simulink model "Embedded_Model_itworks"  (R2024a)
settings: Solver=FixedStepDiscrete  StartTime=0.0  StopTime=Inf  FixedStep=0.002  RelTol=1e-3  EnableMultiTasking=on
values from neighbouring files (symbols this model uses):
  theta_hip_rad = [0 5e-06 2.2e-05 4.9e-05 8.8e-05 0.000137 0.000197 0.000268 0.000349 0.000441 0.000545 0.000657 ... (1200 elements, 1x1200)]    [target_theta_vector.mat]
  theta_knee_rad = [0 -1.2e-05 -4.9e-05 -0.00011 -0.000196 -0.000304 -0.000438 -0.000596 -0.000776 -0.00098 -0.001209 -0.001459 ... (1200 elements, 1x1200)]    [target_theta_vector.mat]
  theta_l1_rad = [0 0 0 0 0 0 0 0 0 0 0 0 ... (1200 elements, 1x1200)]    [target_theta_vector.mat]
undefined symbols (not defined in the file or in its folder): Down, GPTRIP1SEL, TZ1, Up
libraries: c280xlib x10, c2000lib x1, c2837xDlib x1, slpidlib x1, c2802xlib x1
settings Model: ExtModeTrigDuration=8  Creator=The MathWorks, Inc.  LastModifiedBy=wnsgh
settings SolverCC: AllowMultiTaskInputOutput=on  AlgebraicLoopSolver=TrustRegion  AutoInsertRateTranBlk=on  MaxZcPerStep=1
settings OptimizationCC: DefaultUnderspecifiedDataType=single  EnhancedBackFolding=on  PassReuseOutputArgsAs=Individual arguments  MaxStackSize=1024  OptimizeBlockOrder=speed  DifferentSizesBufferReuse=on  OptimizationCustomize=off  DenormalBehavior=FlushToZero  EfficientTunableParamExpr=on
settings DebuggingCC: MultiTaskDSMMsg=none  ParameterTunabilityLossMsg=error  UnconnectedInputMsg=warning  UnconnectedOutputMsg=warning  UnconnectedLineMsg=warning
settings HardwareCC: ProdBitPerChar=16  ProdBitPerInt=16  ProdBitPerPointer=32  ProdBitPerSizeT=32  ProdBitPerPtrDiffT=32  ProdLargestAtomicInteger=Integer  ProdLargestAtomicFloat=None  ProdWordSize=16  ProdLongLongMode=on  ProdHWDeviceType=Texas Instruments->C2000
settings ModelReferenceCC: EnableRefExpFcnMdlSchedulingChecks=on
settings SFSimCC: MATLABDynamicMemAlloc=off
settings RTWCC: Description=Embedded Coder  SystemTargetFile=ert.tlc  HardwareBoard=TI Delfino F28379D LaunchPad  TemplateMakefile=ert_default_tmf  GenerateReport=on  Toolchain=Texas Instruments Code Composer Studio (C2000)  GPUComputeCapability=3.5  DLArmComputeVersion=19.05
settings CodeAppCC: ForceParamTrailComments=on  IgnoreCustomStorageClasses=off  OperatorAnnotations=on  SimulinkDataObjDesc=on  SFDataObjDesc=on  InsertBlockDesc=on
settings ERTTargetCC: CodeReplacementLibrary=TI C28x  ExtModeStaticAllocSize=10000

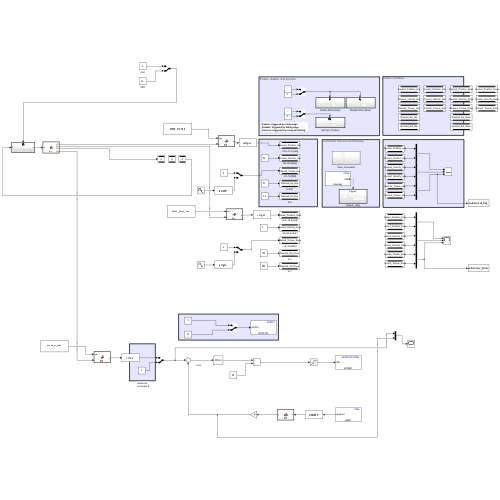
[thumbnail: Simulink's stored preview of the top-level diagram]
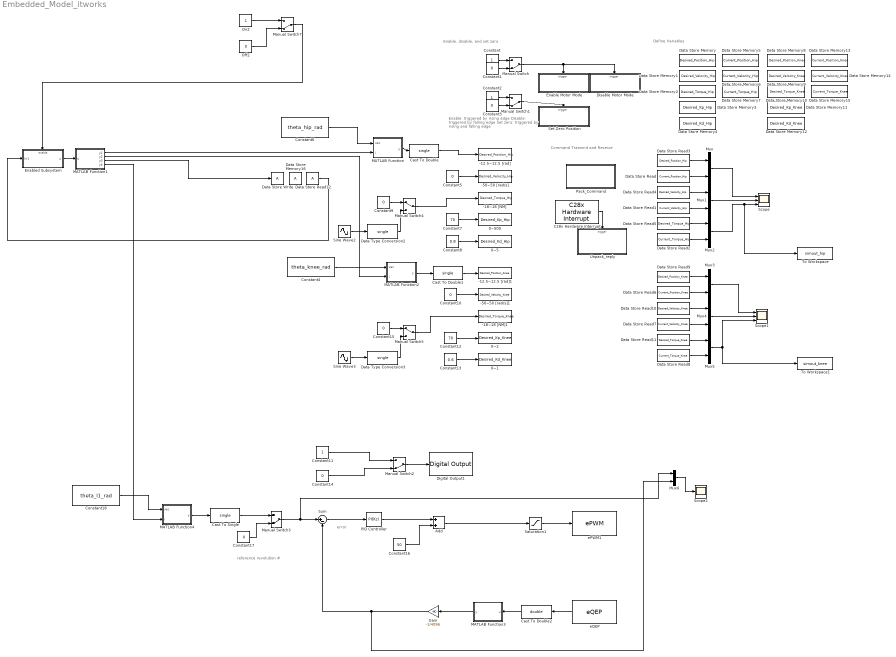
== system Embedded_Model_itworks ==
  note: Enable: triggered by rising edge
      | Disable: triggered by falling edge
      | Set zero: triggered by rising and falling edge
  note: Define Variables
  note: Enable, disable, and set zero
  note: Command Transmit and Receive
  note: reference
      | revolution #
  note: error
  -12.5~12.5 [rad] : DataStoreWrite  DataStoreName=Desired_Position_Hip  IndexOptions=Index vector (dialog)  Indices=1  OutputSizes=1
  -12.5~12.5 [rad]1 : DataStoreWrite  DataStoreName=Desired_Position_Knee  IndexOptions=Index vector (dialog)  Indices=1  OutputSizes=1
  -18~18 [NM] : DataStoreWrite  DataStoreName=Desired_Torque_Hip  IndexOptions=Index vector (dialog)  Indices=1  OutputSizes=1
  -18~18 [NM]1 : DataStoreWrite  DataStoreName=Desired_Torque_Knee  IndexOptions=Index vector (dialog)  Indices=1  OutputSizes=1
  -50~50 [rad/s] : DataStoreWrite  DataStoreName=Desired_Velocity_Hip  IndexOptions=Index vector (dialog)  Indices=1  OutputSizes=1
  -50~50 [rad/s]1 : DataStoreWrite  DataStoreName=Desired_Velocity_Knee  IndexOptions=Index vector (dialog)  Indices=1  OutputSizes=1
  0~1 : DataStoreWrite  DataStoreName=Desired_Kd_Knee  IndexOptions=Index vector (dialog)  Indices=1  OutputSizes=1
  0~2 : DataStoreWrite  DataStoreName=Desired_Kp_Knee  IndexOptions=Index vector (dialog)  Indices=1  OutputSizes=1
  0~5 : DataStoreWrite  DataStoreName=Desired_Kd_Hip  IndexOptions=Index vector (dialog)  Indices=1  OutputSizes=1
  0~500 : DataStoreWrite  DataStoreName=Desired_Kp_Hip  IndexOptions=Index vector (dialog)  Indices=1  OutputSizes=1
  Add : Sum
  C28x Hardware Interrupt : c2000lib/Scheduling/C28x Hardware Interrupt  irqnumbers=[9]  pienumbers=[8]  irqpriorities=[30]  irqpreempts=[1]  showinput=off  dspchiptype=C280X
  Cast To Double : DataTypeConversion  OutDataTypeStr=single  SaturateOnIntegerOverflow=off  RndMeth=Floor
  Cast To Double1 : DataTypeConversion  OutDataTypeStr=single  SaturateOnIntegerOverflow=off  RndMeth=Floor
  Cast To Double2 : DataTypeConversion  OutDataTypeStr=double  SaturateOnIntegerOverflow=off  RndMeth=Floor
  Cast To Single : DataTypeConversion  OutDataTypeStr=single  SaturateOnIntegerOverflow=off  RndMeth=Floor
  Constant : Constant
  Constant{1,3,14,17} (4 alike) : Constant  Value=0
  Constant{5,9..10,15} (4 alike) : Constant  Value=0  OutDataTypeStr=single
  Constant11 : Constant
  Constant12 : Constant  Value=70  OutDataTypeStr=single
  Constant13 : Constant  Value=0.6  OutDataTypeStr=single
  Constant16 : Constant  Value=50
  Constant18 : Constant  Value=theta_l1_rad
  Constant2 : Constant
  Constant4 : Constant  Value=theta_knee_rad
  Constant6 : Constant  Value=theta_hip_rad
  Constant7 : Constant  Value=70  OutDataTypeStr=single
  Constant8 : Constant  Value=0.8  OutDataTypeStr=single
  Data Store Memory : DataStoreMemory  DataStoreName=Desired_Position_Hip  WriteAfterWriteMsg=warning  ShowAdditionalParam=off  OutDataTypeStr=single
  Data Store Memory1 : DataStoreMemory  DataStoreName=Desired_Velocity_Hip  WriteAfterWriteMsg=warning  ShowAdditionalParam=off  OutDataTypeStr=single
  Data Store Memory10 : DataStoreMemory  DataStoreName=Desired_Torque_Knee  WriteAfterWriteMsg=warning  ShowAdditionalParam=off  OutDataTypeStr=single
  Data Store Memory11 : DataStoreMemory  DataStoreName=Desired_Kp_Knee  WriteAfterWriteMsg=warning  ShowAdditionalParam=off  OutDataTypeStr=single
  Data Store Memory12 : DataStoreMemory  DataStoreName=Desired_Kd_Knee  WriteAfterWriteMsg=warning  ShowAdditionalParam=off  OutDataTypeStr=single
  Data Store Memory13 : DataStoreMemory  DataStoreName=Current_Position_Knee  WriteAfterWriteMsg=warning  ShowAdditionalParam=off  OutDataTypeStr=single
  Data Store Memory14 : DataStoreMemory  DataStoreName=Current_Velocity_Knee  WriteAfterWriteMsg=warning  ShowAdditionalParam=off  OutDataTypeStr=single
  Data Store Memory15 : DataStoreMemory  DataStoreName=Current_Torque_Knee  WriteAfterWriteMsg=warning  ShowAdditionalParam=off  OutDataTypeStr=single
  Data Store Memory16 : DataStoreMemory  WriteAfterWriteMsg=warning  ShowAdditionalParam=off
  Data Store Memory2 : DataStoreMemory  DataStoreName=Desired_Torque_Hip  WriteAfterWriteMsg=warning  ShowAdditionalParam=off  OutDataTypeStr=single
  Data Store Memory3 : DataStoreMemory  DataStoreName=Desired_Kp_Hip  WriteAfterWriteMsg=warning  ShowAdditionalParam=off  OutDataTypeStr=single
  Data Store Memory4 : DataStoreMemory  DataStoreName=Desired_Kd_Hip  WriteAfterWriteMsg=warning  ShowAdditionalParam=off  OutDataTypeStr=single
  Data Store Memory5 : DataStoreMemory  DataStoreName=Current_Position_Hip  WriteAfterWriteMsg=warning  ShowAdditionalParam=off  OutDataTypeStr=single
  Data Store Memory6 : DataStoreMemory  DataStoreName=Current_Velocity_Hip  WriteAfterWriteMsg=warning  ShowAdditionalParam=off  OutDataTypeStr=single
  Data Store Memory7 : DataStoreMemory  DataStoreName=Current_Torque_Hip  WriteAfterWriteMsg=warning  ShowAdditionalParam=off  OutDataTypeStr=single
  Data Store Memory8 : DataStoreMemory  DataStoreName=Desired_Position_Knee  WriteAfterWriteMsg=warning  ShowAdditionalParam=off  OutDataTypeStr=single
  Data Store Memory9 : DataStoreMemory  DataStoreName=Desired_Velocity_Knee  WriteAfterWriteMsg=warning  ShowAdditionalParam=off  OutDataTypeStr=single
  Data Store Read : DataStoreRead  DataStoreName=Current_Position_Hip  IndexOptions=Index vector (dialog)  Indices=1  OutputSizes=1
  Data Store Read1 : DataStoreRead  DataStoreName=Current_Velocity_Hip  IndexOptions=Index vector (dialog)  Indices=1  OutputSizes=1
  Data Store Read10 : DataStoreRead  DataStoreName=Desired_Velocity_Knee  IndexOptions=Index vector (dialog)  Indices=1  OutputSizes=1
  Data Store Read11 : DataStoreRead  DataStoreName=Desired_Torque_Knee  IndexOptions=Index vector (dialog)  Indices=1  OutputSizes=1
  Data Store Read12 : DataStoreRead  IndexOptions=Index vector (dialog)  Indices=1  OutputSizes=1
  Data Store Read2 : DataStoreRead  DataStoreName=Current_Torque_Hip  IndexOptions=Index vector (dialog)  Indices=1  OutputSizes=1
  Data Store Read3 : DataStoreRead  DataStoreName=Desired_Position_Hip  IndexOptions=Index vector (dialog)  Indices=1  OutputSizes=1
  Data Store Read4 : DataStoreRead  DataStoreName=Desired_Velocity_Hip  IndexOptions=Index vector (dialog)  Indices=1  OutputSizes=1
  Data Store Read5 : DataStoreRead  DataStoreName=Desired_Torque_Hip  IndexOptions=Index vector (dialog)  Indices=1  OutputSizes=1
  Data Store Read6 : DataStoreRead  DataStoreName=Current_Position_Knee  IndexOptions=Index vector (dialog)  Indices=1  OutputSizes=1
  Data Store Read7 : DataStoreRead  DataStoreName=Current_Velocity_Knee  IndexOptions=Index vector (dialog)  Indices=1  OutputSizes=1
  Data Store Read8 : DataStoreRead  DataStoreName=Current_Torque_Knee  IndexOptions=Index vector (dialog)  Indices=1  OutputSizes=1
  Data Store Read9 : DataStoreRead  DataStoreName=Desired_Position_Knee  IndexOptions=Index vector (dialog)  Indices=1  OutputSizes=1
  Data Store Write : DataStoreWrite  IndexOptions=Index vector (dialog)  Indices=1  OutputSizes=1
  Data Type Conversion2 : DataTypeConversion  OutDataTypeStr=single  SaturateOnIntegerOverflow=off  RndMeth=Floor
  Data Type Conversion3 : DataTypeConversion  OutDataTypeStr=single  SaturateOnIntegerOverflow=off  RndMeth=Floor
  Digital Output1 : c2837xDlib/Digital Output  GPIO_Number=GPIO0~GPIO7  GPIO_Bit0=off  GPIO_BIT0_Toggle=off  GPIO_Bit1=off  GPIO_BIT1_Toggle=off  GPIO_Bit2=off  GPIO_BIT2_Toggle=off  GPIO_Bit3=on  GPIO_BIT3_Toggle=off  GPIO_Bit4=off  GPIO_BIT4_Toggle=off  GPIO_Bit5=off  GPIO_BIT5_Toggle=off  GPIO_Bit6=off  GPIO_BIT6_Toggle=off  GPIO_Bit7=off  GPIO_BIT7_Toggle=off
  Disable Motor Mode : Subsystem
  Enable Motor Mode : Subsystem
  Enabled Subsystem : Subsystem  TreatAsAtomicUnit=on
  Gain : Gain  Gain=-1/4096
  MATLAB Function : MATLAB Function  TreatAsAtomicUnit=on
  MATLAB Function1 : MATLAB Function  TreatAsAtomicUnit=on
  MATLAB Function2 : MATLAB Function  TreatAsAtomicUnit=on
  MATLAB Function3 : MATLAB Function  TreatAsAtomicUnit=on
  MATLAB Function4 : MATLAB Function  TreatAsAtomicUnit=on
  Manual Switch{,1..3,7} (5 alike) : ManualSwitch  CurrentSetting=0
  Manual Switch4 : ManualSwitch
  Manual Switch5 : ManualSwitch
  Mux{,1..6} (7 alike) : Mux  Inputs=2
  Off2 : Constant  Value=0
  On2 : Constant
  PID Controller : slpidlib/PID Controller  Controller=PID  Form=Parallel  TimeDomain=Discrete-time  UseExternalTs=off  SampleTime=-1  IntegratorMethod=Forward Euler  FilterMethod=Forward Euler  ControllerParametersSource=internal  P=70  I=5  UseKiTs=off  D=2  UseExternalDerivativeSource=off  N=100  UseFilter=on  TunerSelectOption=Frequency Response Based  InitialConditionSource=internal  InitialConditionForIntegrator=0  InitialConditionForFilter=0  DifferentiatorICPrevScaledInput=0  ExternalReset=none  TrackingMode=off  Kt=1  LimitOutput=off  SatLimitsSource=internal  UpperSaturationLimit=inf  LowerSaturationLimit=-inf  LinearizeAsGain=on  AntiWindupMode=none  Kb=1  LimitIntegrator=off  UpperIntegratorSaturationLimit=inf  LowerIntegratorSaturationLimit=-inf  POutMin=[]  POutMax=[]  IOutMin=[]  IOutMax=[]  DOutMin=[]  DOutMax=[]  NOutMin=[]  NOutMax=[]  SumOutMin=[]  SumOutMax=[]  SaturationOutMin=[]  SaturationOutMax=[]  PParamMin=[]  PParamMax=[]  IParamMin=[]  IParamMax=[]  DParamMin=[]  DParamMax=[]  NParamMin=[]  NParamMax=[]  KbParamMin=[]  KbParamMax=[]  KtParamMin=[]  KtParamMax=[]  KbOutMin=[]  KbOutMax=[]  KtOutMin=[]  KtOutMax=[]  IntegratorOutMin=[]  IntegratorOutMax=[]  FilterOutMin=[]  FilterOutMax=[]  SumI1OutMin=[]  SumI1OutMax=[]  SumI2OutMin=[]  SumI2OutMax=[]  SumI3OutMin=[]  SumI3OutMax=[]  SumI4OutMin=[]  SumI4OutMax=[]  SumDOutMin=[]  SumDOutMax=[]  DifferentiatorOutMin=[]  DifferentiatorOutMax=[]  FilterDiffOutCoefMin=[]  FilterDiffOutCoefMax=[]  ReciprocalOutMin=[]  ReciprocalOutMax=[]  SumDenOutMin=[]  SumDenOutMax=[]  SumNumOutMin=[]  SumNumOutMax=[]  DivideOutMin=[]  DivideOutMax=[]  UdiffTsProdOutMin=[]  UdiffTsProdOutMax=[]  NTsProdOutMin=[]  NTsProdOutMax=[]  UintegralTsProdOutMin=[]  UintegralTsProdOutMax=[]  UngainTsProdOutMin=[]  UngainTsProdOutMax=[]  ClampingZeroOutDataTypeStr=Inherit: Inherit via back propagation  ClampingZeroOutMin=[]  ClampingZeroOutMax=[]  FilterDenConstantOutDataTypeStr=Inherit: Inherit via back propagation  FilterDenConstantOutMin=[]  FilterDenConstantOutMax=[]  PCopyOutDataTypeStr=Inherit: Inherit via back propagation  PCopyOutMin=[]  PCopyOutMax=[]  NCopyOutDataTypeStr=Inherit: Inherit via back propagation  NCopyOutMin=[]  NCopyOutMax=[]  IntegratorContinuousStateAttributes=''  IntegratorStateMustResolveToSignalObject=off  IntegratorRTWStateStorageClass=Auto  FilterContinuousStateAttributes=''  FilterStateMustResolveToSignalObject=off  FilterRTWStateStorageClass=Auto  ParallelPVariant=InternalParameters  IdealPVariant=Disabled  IVariant=InternalParameters  DVariant=InternalParameters  IntegratorVariant=Discrete  SatVariant=Disabled  AWVariant=Passthrough  PCopyVariant=Disabled  TRVariant=Disabled  FdbkBlocksVariant=Forward  IdealPFdbkVariant=Disabled  SatFdbkVariant=Disabled  DerivativeFilterVariant=ForwardEulerFilter  NVariant=InternalParameters  NCopyVariant=Disabled  FilterICVariant=InternalICsFilter  IntegratorICVariant=InternalICs  ExternalResetVariant=Disabled  TRSumVariant=Passthrough  SumFdbkVariant=Disabled  SumVariant=Sum_PID  TsampFilterVariant=InternalTs  TsampNgainVariant=Passthrough  TsampIntegralVariant=Disabled_SignalSpec  ExternalSaturationOutDataTypeStr=Inherit: Same as second input  DerivativeSourceVariant=ErrorSignal
  Pack_Command : Subsystem
  Saturation1 : Saturate  UpperLimit=90  LowerLimit=10
  Scope : Scope  NumInputPorts=3
  Scope1 : Scope  NumInputPorts=3
  Scope2 : Scope
  Set Zero Position : Subsystem
  Sine Wave2 : Sin  Amplitude=0.5  Frequency=2*pi
  Sine Wave3 : Sin  Amplitude=0.5  Frequency=2*pi
  Sum : Sum  Inputs=|+-
  To Workspace : ToWorkspace  VariableName=simout_hip  SampleTime=-1
      settings: Save2DSignal=2-D array (concatenate along first dimension)
  To Workspace1 : ToWorkspace  VariableName=simout_knee  SampleTime=-1
      settings: Save2DSignal=2-D array (concatenate along first dimension)
  Unpack_reply : Subsystem  ScheduleAs=Aperiodic partition  PartitionName=Unpack_reply
  ePWM1 : c2802xlib/ePWM  PwmType=C2000_Type4  useModule=ePWM1  ePWMxLINKTBPRD=Not Linked  periodUnits=Seconds  timerSource=Specify via dialog  timerPeriod_clk=64000  timerPeriod_sec=0.0001  tbshadow=Counter equals to zero  countingMode=Up-Down  phaseActiveEnable=Disable  phaseDirection=Count down after sync  phaseActive=0  synchronizationEnable=off  dcaevt1Sync=off  dcbevt1Sync=off  synchronizationOption=Disable  dcbevt1SyncOut=off  dcaevt1SyncOut=off  cmpdSyncOut=off  cmpcSyncOut=off  cmpbSyncOut=off  zeroSyncOut=off  swfSyncOut=off  perSynchronizationOption=Counter equals to period (CTR=PRD)  clockPrescale=1  HSclockPrescale=1  enswap=off  ePWMxAStatus=on  ePWMxAactionLogic1=Set  ePWMxAactionLogic2=Clear  ePWMxAactionLogic3=Clear  ePWMxAactionLogic4=Set  ePWMxAactionLogic5=Do nothing  ePWMxAactionLogic6=Do nothing  ePWMxACSFenable=off  ePWMxACSFvalue=Forcing disable  ePWMxASFreload=Zero  ePWMxBStatus=off  ePWMxBactionLogic1=Set  ePWMxBactionLogic2=Clear  ePWMxBactionLogic3=Do nothing  ePWMxBactionLogic4=Do nothing  ePWMxBactionLogic5=Clear  ePWMxBactionLogic6=Set  ePWMxBCSFenable=off  ePWMxBCSFvalue=Forcing disable  ePWMxBSFreload=Zero  ePWNxBOutWay=off  ePWMxLINKCMPA=Not Linked  CMPAUnits=Percentages  CMPASource=Input port  CMPAValue_per=50  CMPAValue_clk=32000  enCMPAshadow=Counter equals to zero (CTR=Zero)  ePWMxLINKCMPB=Not Linked  CMPBUnits=Percentages  CMPBSource=Specify via dialog  CMPBValue_per=50  CMPBValue_clk=32000  enCMPBshadow=Counter equals to zero (CTR=Zero)  ePWMxLINKCMPC=Not Linked  CMPCUnits=Clock cycles  CMPCSource=Specify via dialog  CMPCValue_per=50  CMPCValue_clk=32000  enCMPCshadow=Counter equals to zero (CTR=Zero)  ePWMxLINKCMPD=Not Linked  CMPDUnits=Clock cycles  CMPDSource=Specify via dialog  CMPDValue_per=50  CMPDValue_clk=32000  enCMPDshadow=Counter equals to zero (CTR=Zero)  enableDBePWMxA=off  enableDBePWMxB=off  enhalfcycle=off  DBpolarity=Active high (AH)  DBedgeDelay=Positive  DBSource_ePWMxA=ePWMxA  DBSource_ePWMxB=ePWMxA  DBPeriodUnits=Clock cycles  DBperiodSource=Specify via dialog  REDperiod=0  FEDperiod=0  REDperiod_sec=0  FEDperiod_sec=0  LoadModeDBRED=Immediate without using shadow  LoadModeDBFED=Immediate without using shadow  adcstartModuleA=off  adcrequestEventA=First event  adcstartEventA=Digital Compare Module A Event 1 start of conversion (DCAEVT1.soc)  adcstartEventA_type2=Counter equals to zero (CTR=Zero)  adcstartModuleB=off  adcrequestEventB=First event  adcstartEventB=Counter equals to zero (CTR=Zero)  adcstartEventB_type2=Counter equals to zero (CTR=Zero)  intEn=off  intPrd=First event  intSel=Counter equals to zero (CTR=Zero)  intSel_type2=Counter equals to zero (CTR=Zero)  hrpe=off  enHRPWM=off  HRPWM_LoadMode=Counter equals to period (CTR=PRD)  HRPWM_CTLMode=Duty or Period control mode  HRPWM_EDGMode=Both edge  hrpeb=off  enHRPWMB=off  HRPWM_LoadModeB=Counter equals to zero (CTR=ZERO)  HRPWM_CTLModeB=Duty or Period control mode  HRPWM_EDGModeB=Both edge  enHRDBRED=off  enHRDBFED=off  enSFO=on  enautoconv=on  chopperEnable=off  chopperFrequency=1  chopperFirstwidth=1  chopperDuty=12.5%  tripZonesource=Specify via dialog  tzselOSHT1=off  tzselOSHT2=off  tzselOSHT3=off  tzselOSHT4=off  tzselOSHT5=off  tzselOSHT6=off  tzselOSHDCAEV1=off  tzselOSHDCBEV1=off  tzselCBC1=off  tzselCBC2=off  tzselCBC3=off  tzselCBC4=off  tzselCBC5=off  tzselCBC6=off  tzselCBCDCAEV2=off  tzselCBCDCBEV2=off  enTzOstIntr=off  enTzCbcIntr=off  enTzDCAEVT1Intr=off  enTzDCAEVT2Intr=off  enTzDCBEVT1Intr=off  enTzDCBEVT2Intr=off  tzclrCBCLatch=Counter equals to zero (CTR=Zero)  ePWMxAforced=No action  ePWMxBforced=No action  DCAEVT1forced=No action  DCBEVT1forced=No action  DCAEVT2forced=No action  DCBEVT2forced=No action  dcah=Trip Zone 1 input (TZ1)  dcal=Trip Zone 2 input (TZ2)  dcbh=Trip Zone 1 input (TZ1)  dcbl=Trip Zone 2 input (TZ2)  dcah_type2=GPTRIP1SEL/(TZ1)  dcal_type2=GPTRIP1SEL/(TZ1)  dcbh_type2=GPTRIP1SEL/(TZ1)  dcbl_type2=GPTRIP1SEL/(TZ1)  gendcaevt1=Event disabled  gendcaevt2=Event disabled  gendcbevt1=Event disabled  gendcbevt2=Event disabled  dcaevt1src=DCAEVT1 with sync  dcaevt2src=DCAEVT2 with sync  dcbevt1src=DCBEVT1 with sync  dcbevt2src=DCBEVT2 with sync  pulsesel=Counter equals to zero (CTR=Zero)  blankinv=off  blankoffset=0  blankwidth=0  evsrcsel=Filtered version of DCAEVT1 (DCAEVT1FILT)  encape=off
      settings: LibrarySourceBlock=c2837xDlib/ePWM
  eQEP : c280xlib/eQEP  useModule=eQEP1  pcInputmode=Quadrature-count  externalClockrate=2x resolution: Count the rising/falling edge  swapPolarityselection=Clockwise  qdfOutputport=off  qapPolarityselection=off  qbpPolarityselection=off  qipPolarityselection=off  qspPolarityselection=off  igatePolarityselection=off  sampleTime=-1  pcOutputport=on  pcMaximumvalue=2^24  indexInitializationcheck=off  indexInitializationevent=Rising edge  strobeInitializationcheck=off  strobeInitializationevent=Rising edge  softwareInitializationcheck=off  softwareInitializationsource=Set to init value at start up  softwareInitializationmode=on  pcInitialvalue=2147483648  pcResetmode=Reset on an index event  ieloutputport=off  indexEventlatch=Rising edge  seloutputport=off  strobeEventlatch=Rising edge  pcefOutputport=off  enableEqepcapture=off  qctmrOutputport=off  qcprdOutputport=off  captureTimerprescaler=128  upEventprescaler=128  overflowErrorflag=off  directionErrorflag=off  captureTimerposition=On position counter read  unitTimerperiod=100000000  captureTimerlatch=off  capturePeriodlatch=off  positionCounterlatch=off  soenPolarityselection=off  spselPolarityselection=Index pin is used for sync output  compareValuesource=Specify via dialog  shadowMode=Load on QPOSCNT=0  compareValue=4294967295  syncOutputwidth=1  polaritySyncoutput=Active high  watchdogEnable=off  watchdogTimer=65535  outport1Datatype=auto  outport2Datatype=auto  outport3Datatype=auto  outport4Datatype=auto  outport5Datatype=auto  outport6Datatype=auto  outport7Datatype=auto  outport8Datatype=auto  outport9Datatype=auto  outport10Datatype=auto  outport11Datatype=auto  outport12Datatype=auto  eqepinterrupt_pce=off  eqepinterrupt_qpe=off  eqepinterrupt_qdc=off  eqepinterrupt_wto=off  eqepinterrupt_pcu=off  eqepinterrupt_pco=off  eqepinterrupt_pcr=off  eqepinterrupt_pcm=off  eqepinterrupt_sel=off  eqepinterrupt_iel=off  eqepinterrupt_uto=off  pheOutputport=off  watchdogOutputport=off  outport13Datatype=auto  outport14Datatype=auto
      settings: LibrarySourceBlock=c2837xDlib/eQEP
  wires:
  Data Store Read9/1 -> Mux3/1
  Constant5/1 -> -50~50 [rad/s]/1
  Data Store Read8/1 -> Mux5/2
  Mux1/1 -> Scope/2
  Mux4/1 -> Scope1/2
  Data Store Read7/1 -> Mux4/2
  Constant13/1 -> 0~1/1
  Data Store Read10/1 -> Mux4/1
  Data Store Read11/1 -> Mux5/1
  Data Store Read6/1 -> Mux3/2
  Constant12/1 -> 0~2/1
  Mux5/1 -> To Workspace1/1, Scope1/3
  Constant2/1 -> Manual Switch1/1
  Mux2/1 -> To Workspace/1, Scope/3
  Constant/1 -> Manual Switch/1
  Data Store Read2/1 -> Mux2/2
  Data Store Read/1 -> Mux/2
  Data Store Read3/1 -> Mux/1
  Data Store Read5/1 -> Mux2/1
  Constant10/1 -> -50~50 [rad/s]1/1
  Data Store Read4/1 -> Mux1/1
  Constant7/1 -> 0~500/1
  Data Store Read1/1 -> Mux1/2
  Manual Switch1/1 -> Set Zero Position/Trigger
  Mux3/1 -> Scope1/1
  Constant3/1 -> Manual Switch1/2
  Manual Switch/1 -> Enable Motor Mode/Trigger, Disable Motor Mode/Trigger
  Constant1/1 -> Manual Switch/2
  Constant8/1 -> 0~5/1
  Mux/1 -> Scope/1
  C28x Hardware Interrupt/1 -> Unpack_reply/Trigger
  Sine Wave2/1 -> Data Type Conversion2/1
  Constant9/1 -> Manual Switch4/1
  Data Type Conversion2/1 -> Manual Switch4/2
  Constant15/1 -> Manual Switch5/1
  Data Type Conversion3/1 -> Manual Switch5/2
  Sine Wave3/1 -> Data Type Conversion3/1
  Manual Switch4/1 -> -18~18 [NM]/1
  Manual Switch5/1 -> -18~18 [NM]1/1
  MATLAB Function1/1(y1) -> MATLAB Function/2(i)
  MATLAB Function1/3(y3) -> Data Store Write/1
  Data Store Read12/1 -> Enabled Subsystem/1(In1)
  Enabled Subsystem/1(u) -> MATLAB Function1/1(u)
  Constant6/1 -> MATLAB Function/1(vec)
  Constant4/1 -> MATLAB Function2/1(vec)
  MATLAB Function1/2(y2) -> MATLAB Function2/2(i)
  MATLAB Function/1(y) -> Cast To Double/1
  Cast To Double/1 -> -12.5~12.5 [rad]/1
  MATLAB Function2/1(y) -> Cast To Double1/1
  Cast To Double1/1 -> -12.5~12.5 [rad]1/1
  Cast To Single/1 -> Manual Switch3/1
  Add/1 -> Saturation1/1
  Cast To Double2/1 -> MATLAB Function3/1(u)
  Saturation1/1 -> ePWM1/1
  PID Controller/1 -> Add/1
  Gain/1 -> Mux6/2, Sum/2
  Sum/1 -> PID Controller/1
  MATLAB Function3/1(y) -> Gain/1
  Manual Switch2/1 -> Digital Output1/1
  Constant14/1 -> Manual Switch2/2
  Constant17/1 -> Manual Switch3/2
  eQEP/1 -> Cast To Double2/1
  Manual Switch3/1 -> Mux6/1, Sum/1
  Constant16/1 -> Add/2
  Constant11/1 -> Manual Switch2/1
  Mux6/1 -> Scope2/1
  Constant18/1 -> MATLAB Function4/1(vec)
  MATLAB Function4/1(y) -> Cast To Single/1
  MATLAB Function1/4(y4) -> MATLAB Function4/2(i)
  On2/1 -> Manual Switch7/1
  Off2/1 -> Manual Switch7/2
  Manual Switch7/1 -> Enabled Subsystem/Enable

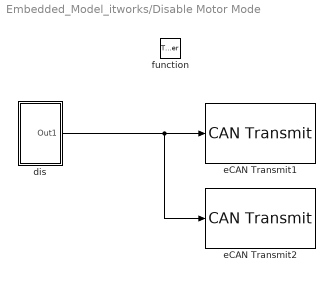
== system Embedded_Model_itworks/Disable Motor Mode ==
  function : TriggerPort  TriggerType=falling  VariantControl=(inherit)
  dis : Subsystem
  eCAN Transmit1 : c280xlib/CAN Transmit  chipFamily=C280x  useModule=CAN_B  mailboxNo=5  messageID=1  messageType=Standard (11-bit identifier)  enableBlockingMode=off  postInterrupt=off  interruptLine=0
  eCAN Transmit2 : c280xlib/CAN Transmit  chipFamily=C280x  useModule=CAN_B  mailboxNo=6  messageID=2  messageType=Standard (11-bit identifier)  enableBlockingMode=off  postInterrupt=off  interruptLine=0
  wires:
  dis/1(Out1) -> eCAN Transmit2/1, eCAN Transmit1/1

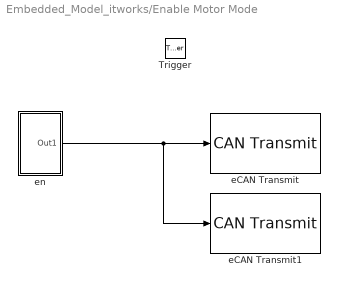
== system Embedded_Model_itworks/Enable Motor Mode ==
  Trigger : TriggerPort  VariantControl=(inherit)  PortDimensions=1
  eCAN Transmit : c280xlib/CAN Transmit  chipFamily=C280x  useModule=CAN_B  mailboxNo=3  messageID=1  messageType=Standard (11-bit identifier)  enableBlockingMode=off  postInterrupt=off  interruptLine=0
  eCAN Transmit1 : c280xlib/CAN Transmit  chipFamily=C280x  useModule=CAN_B  mailboxNo=4  messageID=2  messageType=Standard (11-bit identifier)  enableBlockingMode=off  postInterrupt=off  interruptLine=0
  en : Subsystem
  wires:
  en/1(Out1) -> eCAN Transmit1/1, eCAN Transmit/1

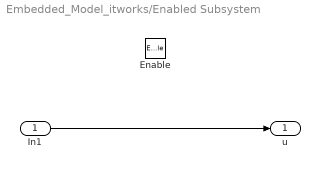
== system Embedded_Model_itworks/Enabled Subsystem ==
  In1 : Inport
  Enable : EnablePort
  u : Outport
  wires:
  In1/1 -> u/1

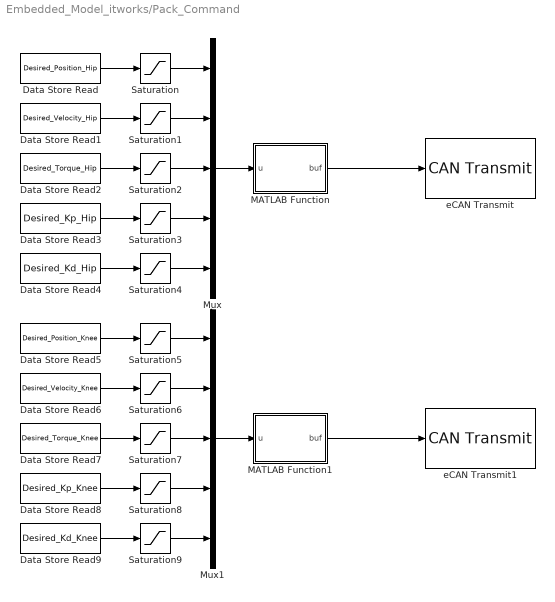
== system Embedded_Model_itworks/Pack_Command ==
  Data Store Read : DataStoreRead  DataStoreName=Desired_Position_Hip  IndexOptions=Index vector (dialog)  Indices=1  OutputSizes=1
  Data Store Read1 : DataStoreRead  DataStoreName=Desired_Velocity_Hip  IndexOptions=Index vector (dialog)  Indices=1  OutputSizes=1
  Data Store Read2 : DataStoreRead  DataStoreName=Desired_Torque_Hip  IndexOptions=Index vector (dialog)  Indices=1  OutputSizes=1
  Data Store Read3 : DataStoreRead  DataStoreName=Desired_Kp_Hip  IndexOptions=Index vector (dialog)  Indices=1  OutputSizes=1
  Data Store Read4 : DataStoreRead  DataStoreName=Desired_Kd_Hip  IndexOptions=Index vector (dialog)  Indices=1  OutputSizes=1
  Data Store Read5 : DataStoreRead  DataStoreName=Desired_Position_Knee  IndexOptions=Index vector (dialog)  Indices=1  OutputSizes=1
  Data Store Read6 : DataStoreRead  DataStoreName=Desired_Velocity_Knee  IndexOptions=Index vector (dialog)  Indices=1  OutputSizes=1
  Data Store Read7 : DataStoreRead  DataStoreName=Desired_Torque_Knee  IndexOptions=Index vector (dialog)  Indices=1  OutputSizes=1
  Data Store Read8 : DataStoreRead  DataStoreName=Desired_Kp_Knee  IndexOptions=Index vector (dialog)  Indices=1  OutputSizes=1
  Data Store Read9 : DataStoreRead  DataStoreName=Desired_Kd_Knee  IndexOptions=Index vector (dialog)  Indices=1  OutputSizes=1
  MATLAB Function : MATLAB Function  TreatAsAtomicUnit=on
  MATLAB Function1 : MATLAB Function  TreatAsAtomicUnit=on
  Mux : Mux  Inputs=5
  Mux1 : Mux  Inputs=5
  Saturation : Saturate  UpperLimit=12.5  LowerLimit=-12.5
  Saturation1 : Saturate  UpperLimit=45  LowerLimit=-45
  Saturation2 : Saturate  UpperLimit=15  LowerLimit=-15
  Saturation3 : Saturate  UpperLimit=500  LowerLimit=0
  Saturation4 : Saturate  UpperLimit=5  LowerLimit=0
  Saturation5 : Saturate  UpperLimit=12.5  LowerLimit=-12.5
  Saturation6 : Saturate  UpperLimit=45  LowerLimit=-45
  Saturation7 : Saturate  UpperLimit=15  LowerLimit=-15
  Saturation8 : Saturate  UpperLimit=500  LowerLimit=0
  Saturation9 : Saturate  UpperLimit=5  LowerLimit=0
  eCAN Transmit : c280xlib/CAN Transmit  chipFamily=C280x  useModule=CAN_B  mailboxNo=1  messageID=1  messageType=Standard (11-bit identifier)  enableBlockingMode=off  postInterrupt=off  interruptLine=0
  eCAN Transmit1 : c280xlib/CAN Transmit  chipFamily=C280x  useModule=CAN_B  mailboxNo=2  messageID=bin2dec('00000000010')  messageType=Standard (11-bit identifier)  enableBlockingMode=off  postInterrupt=off  interruptLine=0
  wires:
  Data Store Read/1 -> Saturation/1
  Data Store Read1/1 -> Saturation1/1
  Data Store Read2/1 -> Saturation2/1
  Data Store Read3/1 -> Saturation3/1
  Data Store Read4/1 -> Saturation4/1
  Saturation/1 -> Mux/1
  Saturation1/1 -> Mux/2
  Saturation2/1 -> Mux/3
  Saturation3/1 -> Mux/4
  Saturation4/1 -> Mux/5
  Mux/1 -> MATLAB Function/1(u)
  MATLAB Function/1(buf) -> eCAN Transmit/1
  Data Store Read8/1 -> Saturation8/1
  Data Store Read7/1 -> Saturation7/1
  Data Store Read5/1 -> Saturation5/1
  Data Store Read6/1 -> Saturation6/1
  Saturation6/1 -> Mux1/2
  Saturation5/1 -> Mux1/1
  MATLAB Function1/1(buf) -> eCAN Transmit1/1
  Saturation8/1 -> Mux1/4
  Mux1/1 -> MATLAB Function1/1(u)
  Saturation7/1 -> Mux1/3
  Saturation9/1 -> Mux1/5
  Data Store Read9/1 -> Saturation9/1

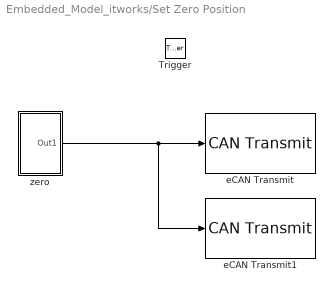
== system Embedded_Model_itworks/Set Zero Position ==
  Trigger : TriggerPort  TriggerType=either  VariantControl=(inherit)  PortDimensions=1
  eCAN Transmit : c280xlib/CAN Transmit  chipFamily=C280x  useModule=CAN_B  mailboxNo=7  messageID=1  messageType=Standard (11-bit identifier)  enableBlockingMode=off  postInterrupt=off  interruptLine=0
  eCAN Transmit1 : c280xlib/CAN Transmit  chipFamily=C280x  useModule=CAN_B  mailboxNo=8  messageID=2  messageType=Standard (11-bit identifier)  enableBlockingMode=off  postInterrupt=off  interruptLine=0
  zero : Subsystem
  wires:
  zero/1(Out1) -> eCAN Transmit1/1, eCAN Transmit/1

== system Embedded_Model_itworks/Unpack_reply ==
  Trigger : TriggerPort  TriggerType=function-call  VariantControl=(inherit)  PortDimensions=1
  Subsystem : Subsystem
  eCAN Receive : c280xlib/CAN Receive  chipFamily=C280x  useModule=CAN_B  mailboxNo=0  messageID=0  messageType=Standard (11-bit identifier)  enableAcceptanceFiltering=on  messageIDMask=bin2dec('00000000001')  sampleTime=-1  dataType=uint8  outputAction=Output last received values  initValue=0  outputMessageID=off  outputMessageLength=off  outputMessageTimeStamp=off  postInterrupt=on  interruptLine=1
  wires:
  eCAN Receive/2 -> Subsystem/1(message1)
  eCAN Receive/1 -> Subsystem/Trigger

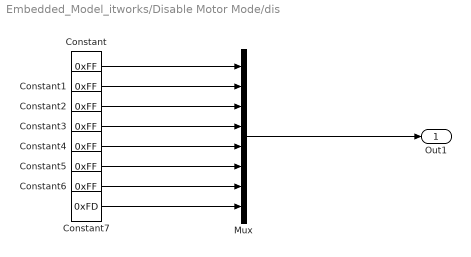
== system Embedded_Model_itworks/Disable Motor Mode/dis ==
  Constant{,1..6} (7 alike) : Constant  Value=0xFF  SampleTime=-1
  Constant7 : Constant  Value=0xFD  SampleTime=-1
  Mux : Mux  Inputs=8
  Out1 : Outport
  wires:
  Mux/1 -> Out1/1
  Constant4/1 -> Mux/5
  Constant1/1 -> Mux/2
  Constant3/1 -> Mux/4
  Constant5/1 -> Mux/6
  Constant/1 -> Mux/1
  Constant6/1 -> Mux/7
  Constant2/1 -> Mux/3
  Constant7/1 -> Mux/8

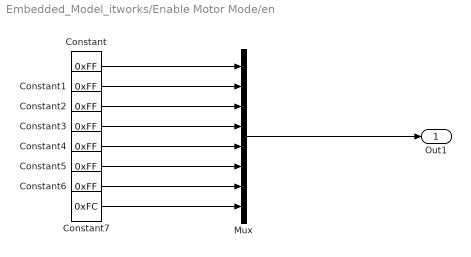
== system Embedded_Model_itworks/Enable Motor Mode/en ==
  Constant{,1..6} (7 alike) : Constant  Value=0xFF  SampleTime=-1
  Constant7 : Constant  Value=0xFC  SampleTime=-1
  Mux : Mux  Inputs=8
  Out1 : Outport
  wires:
  Constant7/1 -> Mux/8
  Constant2/1 -> Mux/3
  Constant6/1 -> Mux/7
  Constant/1 -> Mux/1
  Constant5/1 -> Mux/6
  Constant3/1 -> Mux/4
  Constant1/1 -> Mux/2
  Constant4/1 -> Mux/5
  Mux/1 -> Out1/1

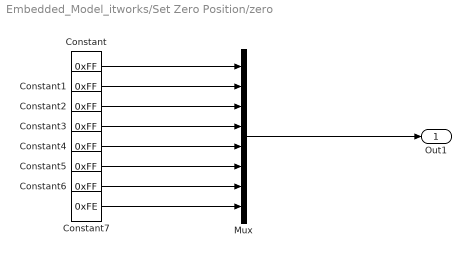
== system Embedded_Model_itworks/Set Zero Position/zero ==
  Constant{,1..6} (7 alike) : Constant  Value=0xFF  SampleTime=-1
  Constant7 : Constant  Value=0xFE  SampleTime=-1
  Mux : Mux  Inputs=8
  Out1 : Outport
  wires:
  Mux/1 -> Out1/1
  Constant4/1 -> Mux/5
  Constant1/1 -> Mux/2
  Constant3/1 -> Mux/4
  Constant5/1 -> Mux/6
  Constant/1 -> Mux/1
  Constant6/1 -> Mux/7
  Constant2/1 -> Mux/3
  Constant7/1 -> Mux/8

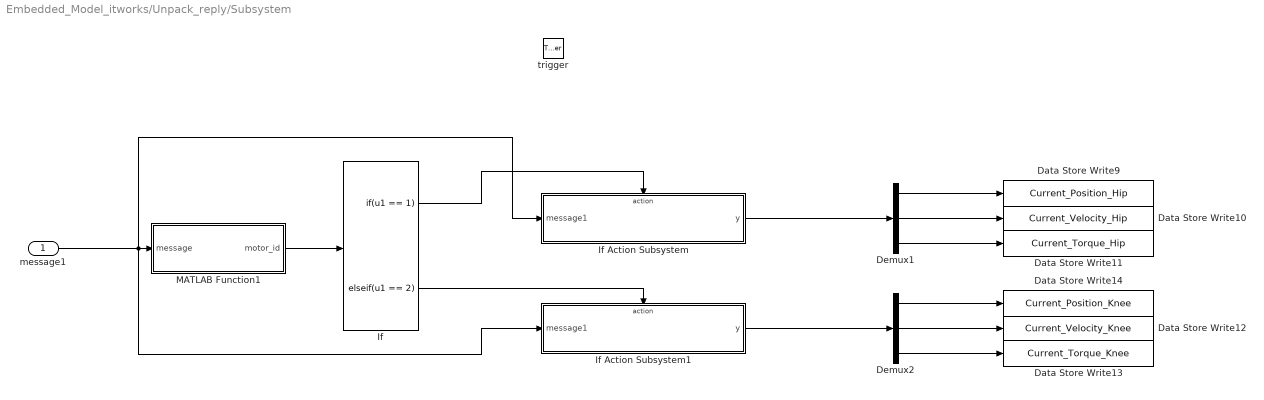
== system Embedded_Model_itworks/Unpack_reply/Subsystem ==
  message1 : Inport
  trigger : TriggerPort  TriggerType=function-call  AsynchronousFunction=on  FunctionName=fcn_async  FunctionVisibility=port  ScopeName=prtscopename  VariantControl=(inherit)  InitialTriggerSignalState=zero
  Data Store Write10 : DataStoreWrite  DataStoreName=Current_Velocity_Hip  IndexOptions=Index vector (dialog)  Indices=1  OutputSizes=1
  Data Store Write11 : DataStoreWrite  DataStoreName=Current_Torque_Hip  IndexOptions=Index vector (dialog)  Indices=1  OutputSizes=1
  Data Store Write12 : DataStoreWrite  DataStoreName=Current_Velocity_Knee  IndexOptions=Index vector (dialog)  Indices=1  OutputSizes=1
  Data Store Write13 : DataStoreWrite  DataStoreName=Current_Torque_Knee  IndexOptions=Index vector (dialog)  Indices=1  OutputSizes=1
  Data Store Write14 : DataStoreWrite  DataStoreName=Current_Position_Knee  IndexOptions=Index vector (dialog)  Indices=1  OutputSizes=1
  Data Store Write9 : DataStoreWrite  DataStoreName=Current_Position_Hip  IndexOptions=Index vector (dialog)  Indices=1  OutputSizes=1
  Demux1 : Demux  Outputs=3
  Demux2 : Demux  Outputs=3
  If : If  IfExpression=u1 == 1  ElseIfExpressions=u1 == 2  ShowElse=off
  If Action Subsystem : Subsystem  TreatAsAtomicUnit=on
  If Action Subsystem1 : Subsystem  TreatAsAtomicUnit=on
  MATLAB Function1 : MATLAB Function  TreatAsAtomicUnit=on
  wires:
  message1/1 -> If Action Subsystem/1(message1), MATLAB Function1/1(message), If Action Subsystem1/1(message1)
  MATLAB Function1/1(motor_id) -> If/1
  If/2 -> If Action Subsystem1/Action
  If/1 -> If Action Subsystem/Action
  Demux1/1 -> Data Store Write9/1
  Demux1/2 -> Data Store Write10/1
  Demux1/3 -> Data Store Write11/1
  If Action Subsystem/1(y) -> Demux1/1
  If Action Subsystem1/1(y) -> Demux2/1
  Demux2/1 -> Data Store Write14/1
  Demux2/3 -> Data Store Write13/1
  Demux2/2 -> Data Store Write12/1

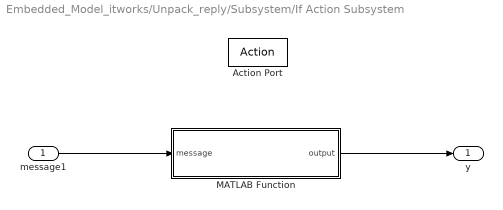
== system Embedded_Model_itworks/Unpack_reply/Subsystem/If Action Subsystem ==
  message1 : Inport
  Action Port : ActionPort  ActionPortLabel=if(u1 == 1)
  MATLAB Function : MATLAB Function  TreatAsAtomicUnit=on
  y : Outport
  wires:
  message1/1 -> MATLAB Function/1(message)
  MATLAB Function/1(output) -> y/1

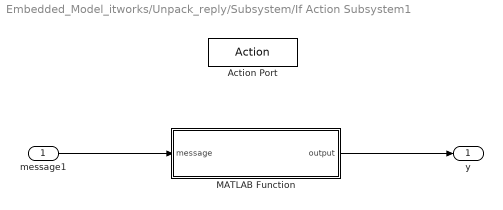
== system Embedded_Model_itworks/Unpack_reply/Subsystem/If Action Subsystem1 ==
  message1 : Inport
  Action Port : ActionPort  ActionPortLabel=elseif(u1 == 2)
  MATLAB Function : MATLAB Function  TreatAsAtomicUnit=on
  y : Outport
  wires:
  message1/1 -> MATLAB Function/1(message)
  MATLAB Function/1(output) -> y/1

== matlab function Embedded_Model_itworks/MATLAB Function ==
  data: vec input; y output; i input
function y = fcn(vec, i)
%#codegen

i = mod(i, length(vec)) + 1; 

y = vec(i);

== matlab function Embedded_Model_itworks/Pack_Command/MATLAB Function ==
  data: u input; buf output
function buf  = fcn(u)
buf = uint8(zeros(1,8));
upos = uint16(((u(1)+12.5)*65535.0/25));
uvel = uint16(((u(2)+45)*4095.0/90));
utor = uint16(((u(3)+15)*4095.0/30));
ukp = uint16(((u(4))*4095.0/500));
ukd = uint16(((u(5))*4095.0/5));

buf(1) = bitshift(upos,-8,'uint16');                                       
buf(2) = bitand(upos, uint16(255),'uint16');   
buf(3) = bitshift(uvel,-4,'uint16');
buf(4) = bitor(bitshift(bitand(uvel, uint16(15),'uint16'),4,'uint16'), bitshift(ukp,-8,'uint16'),'uint16');
buf(5) = bitand(ukp, uint16(255),'uint16');
buf(6) = bitshift(ukd,-4,'uint16');
buf(7) = bitor(bitshift(bitand(ukd , uint16(15),'uint16'),4,'uint16'), bitshift(utor,-8,'uint16'),'uint16');
buf(8) = bitand(utor, uint16(255),'uint16');

== matlab function Embedded_Model_itworks/Pack_Command/MATLAB Function1 ==
  data: u input; buf output
function buf  = fcn(u)
buf = uint8(zeros(1,8));
upos = uint16(((u(1)+12.5)*65535.0/25));
uvel = uint16(((u(2)+45)*4095.0/90));
utor = uint16(((u(3)+15)*4095.0/30));
ukp = uint16(((u(4))*4095.0/500));
ukd = uint16(((u(5))*4095.0/5));

buf(1) = bitshift(upos,-8,'uint16');                                       
buf(2) = bitand(upos, uint16(255),'uint16');   
buf(3) = bitshift(uvel,-4,'uint16');
buf(4) = bitor(bitshift(bitand(uvel, uint16(15),'uint16'),4,'uint16'), bitshift(ukp,-8,'uint16'),'uint16');
buf(5) = bitand(ukp, uint16(255),'uint16');
buf(6) = bitshift(ukd,-4,'uint16');
buf(7) = bitor(bitshift(bitand(ukd , uint16(15),'uint16'),4,'uint16'), bitshift(utor,-8,'uint16'),'uint16');
buf(8) = bitand(utor, uint16(255),'uint16');

== matlab function Embedded_Model_itworks/Unpack_reply/Subsystem/MATLAB Function1 ==
  data: message input; motor_id output
function motor_id = fcn(message)
message = uint16(message);
motor_id = message(1);

== matlab function Embedded_Model_itworks/Unpack_reply/Subsystem/If Action Subsystem/MATLAB Function ==
  data: message input; output output
function output  = Hip_motor(message)
output = single(zeros(1,3));
message = uint16(message);
uintpos = bitor(bitshift(message(2),8,'uint16'),message(3),'uint16');
uintvel = bitor(bitshift(message(4),4,'uint16'), bitshift(message(5),-4,'uint16'),'uint16');
tintvel = bitor(bitshift(bitand(message(5),uint16(15),'uint16'),8,'uint16') , message(6),'uint16');

output(1) = single(uintpos)*25/65535.0 -12.5;
output(2) = single(uintvel)*90/4095.0 -45;
output(3) = single(tintvel)*30/4095.0 -15;

== matlab function Embedded_Model_itworks/Unpack_reply/Subsystem/If Action Subsystem1/MATLAB Function ==
  data: message input; output output
function output  = Knee_motor(message)
output = single(zeros(1,3));
message = uint16(message);
uintpos = bitor(bitshift(message(2),8,'uint16'),message(3),'uint16');
uintvel = bitor(bitshift(message(4),4,'uint16'), bitshift(message(5),-4,'uint16'),'uint16');
tintvel = bitor(bitshift(bitand(message(5),uint16(15),'uint16'),8,'uint16') , message(6),'uint16');

output(1) = single(uintpos)*25/65535.0 -12.5;
output(2) = single(uintvel)*90/4095.0 -45;
output(3) = single(tintvel)*30/4095.0 -15;

== matlab function Embedded_Model_itworks/MATLAB Function1 ==
  data: u input; y1 output; y2 output; y3 output; y4 output
function [y1, y2, y3, y4] = fcn(u)
%#codegen
u = u+1;

y1 = u;
y2 = u;
y3 = u;
y4 = u;

== matlab function Embedded_Model_itworks/MATLAB Function2 ==
  data: vec input; y output; i input
function y = fcn(vec, i)
%#codegen

i = mod(i, length(vec)) + 1; 

y = vec(i);

== matlab function Embedded_Model_itworks/MATLAB Function3 ==
  data: u input; y output
function y = fcn(u)

if u>2^20
    y=-2^24+u;
else
    y=u;
end

== matlab function Embedded_Model_itworks/MATLAB Function4 ==
  data: vec input; y output; i input
function y = fcn(vec, i)
%#codegen

i = mod(i, length(vec)) + 1; 

y = vec(i);
